simulink model "mrefrobotarm_modified_previous_y_previous_u_previous_ref"  (R2018b)
settings: Solver=FixedStepAuto  StartTime=0.0  StopTime=10  RelTol=1e-3  AbsTol=1e-6
undefined symbols (not defined in the file or in its folder): options, sfunxy2
libraries: neural x949, simulink x1
(part 12 of 31)

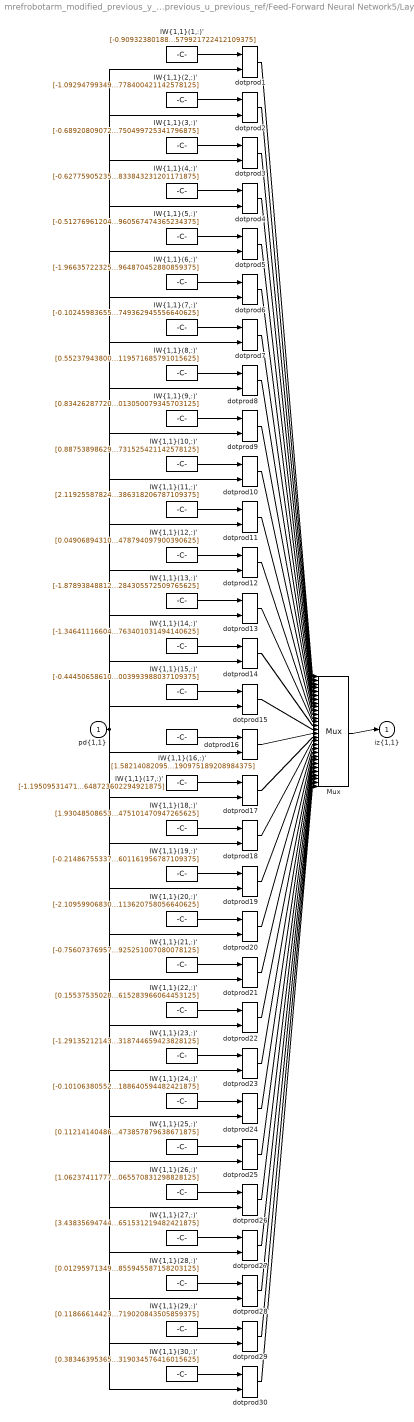
== system mrefrobotarm_modified_previous_y_previous_u_previous_ref/Feed-Forward Neural Network5/Layer 1/IW{1,1} ==
  "pd{1,1}" : Inport  PortDimensions=10
      mask Display: e = 0.06;c1 = [120 230 180]/255;c2 = ([120 230 180]+0)/(256+128);c3 = ([120 230 180]+128)/(256+128);patch([0 1 1 0],[0 0 1 1],c1);patch([0 1 1 1-e 1-e 0+e],[0 0 1 1-e 0+e 0+e],c2);patch([0 0 1 1-e 0+e 0+e],[0 1 1 1-e 1-e 0+e],c3);plot([0 1 1 0 0],[0 0 1 1 0]);
  "IW{1,1}(1,:)'" : Constant  Value=[-0.90932380188037520429844562386278994381427764892578125;0.76371033894988615831067590988823212683200836181640625;0.511083989829526519343971813214011490345001220703125;1.0944032703019865859772608018829487264156341552734375;0.0136695027619473281899065142397375893779098987579345703125;0.1974163924613260012730364678645855747163295745849609375;0.464743606324651781225298918798216618597507476806640625;-0.1561130566172034550564973187647410668432712554931640625;-0.5876780806125221356950305562349967658519744873046875;-0.323235939703412744616883855997002683579921722412109375]
      mask Display: e = 0.06;c1 = [120 150 230]/255;c2 = ([120 150 230]+0)/383;c3 = ([120 150 230]+128)/383;patch([0 1 1 0],[0 0 1 1],c1);patch([0 1 1 1-e 1-e 0+e],[0 0 1 1-e 0+e 0+e],c2);patch([0 0 1 1-e 0+e 0+e],[0 1 1 1-e 1-e 0+e],c3);plot([0 1 1 0 0],[0 0 1 1 0]);disp('Weights');
  "IW{1,1}(10,:)'" : Constant  Value=[0.887538986299241994260000865324400365352630615234375;-1.2998333260689995949377362194354645907878875732421875;0.6289189474694139025956474142731167376041412353515625;0.03883094077027136881152813430162495933473110198974609375;-0.63589794379239228394595784266130067408084869384765625;-0.146677513818444904547533269578707404434680938720703125;-0.313067428723999674478051247206167317926883697509765625;-0.0115715976737959906628372408476934651844203472137451171875;0.42402408377306699538422662953962571918964385986328125;0.1108860373607776228510601868038065731525421142578125]
      mask Display: e = 0.06;c1 = [120 150 230]/255;c2 = ([120 150 230]+0)/383;c3 = ([120 150 230]+128)/383;patch([0 1 1 0],[0 0 1 1],c1);patch([0 1 1 1-e 1-e 0+e],[0 0 1 1-e 0+e 0+e],c2);patch([0 0 1 1-e 0+e 0+e],[0 1 1 1-e 1-e 0+e],c3);plot([0 1 1 0 0],[0 0 1 1 0]);disp('Weights');
  "IW{1,1}(11,:)'" : Constant  Value=[2.119255878248722080314792037825100123882293701171875;-0.7549499748038221991208729377831332385540008544921875;-1.11661451283914647802930630859918892383575439453125;-0.398157577160634323920618271586135961115360260009765625;-1.13162667022485319279212490073405206203460693359375;0.80435012572452035950476556536159478127956390380859375;0.7029651111174974875694942966219969093799591064453125;-0.257844369723556621210036610136739909648895263671875;-0.1686892089893979040926552670498494990170001983642578125;-0.190349557734720453705534737309790216386318206787109375]
      mask Display: e = 0.06;c1 = [120 150 230]/255;c2 = ([120 150 230]+0)/383;c3 = ([120 150 230]+128)/383;patch([0 1 1 0],[0 0 1 1],c1);patch([0 1 1 1-e 1-e 0+e],[0 0 1 1-e 0+e 0+e],c2);patch([0 0 1 1-e 0+e 0+e],[0 1 1 1-e 1-e 0+e],c3);plot([0 1 1 0 0],[0 0 1 1 0]);disp('Weights');
  "IW{1,1}(12,:)'" : Constant  Value=[0.049068943101151452079733417122042737901210784912109375;-1.482782182940682869087822837173007428646087646484375;1.5668343168077765170664861216209828853607177734375;-0.318943372517797529841487857993342913687229156494140625;-0.545573934759136847105764900334179401397705078125;1.1430644568824648299454338484792970120906829833984375;-0.467368252058762478906572823689202778041362762451171875;-0.0230694534923694162531493390133618959225714206695556640625;0.07801593551157563755094059843031573109328746795654296875;0.0214066078871634514479982414059122675098478794097900390625]
      mask Display: e = 0.06;c1 = [120 150 230]/255;c2 = ([120 150 230]+0)/383;c3 = ([120 150 230]+128)/383;patch([0 1 1 0],[0 0 1 1],c1);patch([0 1 1 1-e 1-e 0+e],[0 0 1 1-e 0+e 0+e],c2);patch([0 0 1 1-e 0+e 0+e],[0 1 1 1-e 1-e 0+e],c3);plot([0 1 1 0 0],[0 0 1 1 0]);disp('Weights');
  "IW{1,1}(13,:)'" : Constant  Value=[-1.8789384881240140945379835102357901632785797119140625;3.441410048030609569735815966851077973842620849609375;-1.471086522236758842296922011882998049259185791015625;-0.14898768444497323404362987275817431509494781494140625;-0.399106474358735419105670416684006340801715850830078125;0.6532412791866761825332332591642625629901885986328125;-0.38852173803112322048036730848252773284912109375;0.0032598771438785306177321476894803709001280367374420166015625;-0.01042637952650987860636622173160503734834492206573486328125;0.101455793098639779348246747758821584284305572509765625]
      mask Display: e = 0.06;c1 = [120 150 230]/255;c2 = ([120 150 230]+0)/383;c3 = ([120 150 230]+128)/383;patch([0 1 1 0],[0 0 1 1],c1);patch([0 1 1 1-e 1-e 0+e],[0 0 1 1-e 0+e 0+e],c2);patch([0 0 1 1-e 0+e 0+e],[0 1 1 1-e 1-e 0+e],c3);plot([0 1 1 0 0],[0 0 1 1 0]);disp('Weights');
  "IW{1,1}(14,:)'" : Constant  Value=[-1.3464111660412154680699359232676215469837188720703125;-1.1074716408539320156023677554912865161895751953125;0.2010424729824872580596917259754263795912265777587890625;0.92341948049771682693886987181031145155429840087890625;1.246938309743069961399442036054097115993499755859375;0.01085945570533902553023164472278949688188731670379638671875;-0.81735505804402286411658451470430009067058563232421875;-0.1492403379165857801869066179278888739645481109619140625;-0.26249705798296785186352053642622195184230804443359375;-0.1124250257004068276334152187700965441763401031494140625]
      mask Display: e = 0.06;c1 = [120 150 230]/255;c2 = ([120 150 230]+0)/383;c3 = ([120 150 230]+128)/383;patch([0 1 1 0],[0 0 1 1],c1);patch([0 1 1 1-e 1-e 0+e],[0 0 1 1-e 0+e 0+e],c2);patch([0 0 1 1-e 0+e 0+e],[0 1 1 1-e 1-e 0+e],c3);plot([0 1 1 0 0],[0 0 1 1 0]);disp('Weights');
  "IW{1,1}(15,:)'" : Constant  Value=[-0.444506586108001811030732142171473242342472076416015625;-0.97492464854400318063909480770234949886798858642578125;-0.13235530416492380378912230298737995326519012451171875;0.041227831087679085719788218966641579754650592803955078125;0.302266181113509058153709929683827795088291168212890625;0.78147258701436339567436561992508359253406524658203125;-0.95056085210709528876549256892758421599864959716796875;-0.12105152846243098785361524960535462014377117156982421875;-0.25617381118761428648866740331868641078472137451171875;-0.1020694078831504147952813355004764162003993988037109375]
      mask Display: e = 0.06;c1 = [120 150 230]/255;c2 = ([120 150 230]+0)/383;c3 = ([120 150 230]+128)/383;patch([0 1 1 0],[0 0 1 1],c1);patch([0 1 1 1-e 1-e 0+e],[0 0 1 1-e 0+e 0+e],c2);patch([0 0 1 1-e 0+e 0+e],[0 1 1 1-e 1-e 0+e],c3);plot([0 1 1 0 0],[0 0 1 1 0]);disp('Weights');
  "IW{1,1}(16,:)'" : Constant  Value=[1.5821408209558025514951395962270908057689666748046875;-0.06572990373471408742656052481834194622933864593505859375;-0.315110468167437096642657934353337623178958892822265625;-0.546724857613621662011382795753888785839080810546875;0.6203138051412249165394996452960185706615447998046875;-0.313776979421296953187692224673810414969921112060546875;0.757180165723499332131041228421963751316070556640625;-0.54836876706250758939376055423053912818431854248046875;-0.701850548599278756256580891204066574573516845703125;-0.5565611120524296406841813222854398190975189208984375]
      mask Display: e = 0.06;c1 = [120 150 230]/255;c2 = ([120 150 230]+0)/383;c3 = ([120 150 230]+128)/383;patch([0 1 1 0],[0 0 1 1],c1);patch([0 1 1 1-e 1-e 0+e],[0 0 1 1-e 0+e 0+e],c2);patch([0 0 1 1-e 0+e 0+e],[0 1 1 1-e 1-e 0+e],c3);plot([0 1 1 0 0],[0 0 1 1 0]);disp('Weights');
  "IW{1,1}(17,:)'" : Constant  Value=[-1.1950953147174991908485708336229436099529266357421875;2.3757652564865896493984109838493168354034423828125;-0.38308523924205239996609861918841488659381866455078125;-0.96383528447031319164040041869156993925571441650390625;0.2203039003468626744197678135606111027300357818603515625;-0.497348839684495114266127302471431903541088104248046875;0.1697163099235504402084728781119338236749172210693359375;-0.04046984692262479976765376932235085405409336090087890625;0.2877799138689625113585179860820062458515167236328125;-0.232984678848339121781663152432884089648723602294921875]
      mask Display: e = 0.06;c1 = [120 150 230]/255;c2 = ([120 150 230]+0)/383;c3 = ([120 150 230]+128)/383;patch([0 1 1 0],[0 0 1 1],c1);patch([0 1 1 1-e 1-e 0+e],[0 0 1 1-e 0+e 0+e],c2);patch([0 0 1 1-e 0+e 0+e],[0 1 1 1-e 1-e 0+e],c3);plot([0 1 1 0 0],[0 0 1 1 0]);disp('Weights');
  "IW{1,1}(18,:)'" : Constant  Value=[1.930485086537676142626196451601572334766387939453125;-1.2072210605310542685941754825762473046779632568359375;-0.711007077704297163478486254462040960788726806640625;-0.2130863010885823694007257245175424031913280487060546875;-0.40379224197537089136034182956791482865810394287109375;1.7657478700875628430111419220338575541973114013671875;-1.5367708627335885385178926298976875841617584228515625;0.2230269588249802203971938752147252671420574188232421875;0.28436213533471310643818696917151100933551788330078125;0.565124166666441940520826392457820475101470947265625]
      mask Display: e = 0.06;c1 = [120 150 230]/255;c2 = ([120 150 230]+0)/383;c3 = ([120 150 230]+128)/383;patch([0 1 1 0],[0 0 1 1],c1);patch([0 1 1 1-e 1-e 0+e],[0 0 1 1-e 0+e 0+e],c2);patch([0 0 1 1-e 0+e 0+e],[0 1 1 1-e 1-e 0+e],c3);plot([0 1 1 0 0],[0 0 1 1 0]);disp('Weights');
  "IW{1,1}(19,:)'" : Constant  Value=[-0.21486755337977625490708533106953836977481842041015625;0.395584246940376804690941980879870243370532989501953125;-0.2253224646851052781482138698265771381556987762451171875;0.040212706119560938378132419757093884982168674468994140625;0.63784511537261978642021631458192132413387298583984375;1.05208490378944485854617596487514674663543701171875;-1.9098567669794672685412706414354033768177032470703125;-0.421676708484349571648408527835272252559661865234375;0.83670495443842762828268178054713644087314605712890625;0.371391406764616183178162600597715936601161956787109375]
      mask Display: e = 0.06;c1 = [120 150 230]/255;c2 = ([120 150 230]+0)/383;c3 = ([120 150 230]+128)/383;patch([0 1 1 0],[0 0 1 1],c1);patch([0 1 1 1-e 1-e 0+e],[0 0 1 1-e 0+e 0+e],c2);patch([0 0 1 1-e 0+e 0+e],[0 1 1 1-e 1-e 0+e],c3);plot([0 1 1 0 0],[0 0 1 1 0]);disp('Weights');
  "IW{1,1}(2,:)'" : Constant  Value=[-1.0929479934920554029531558626331388950347900390625;-0.9110333206059608723847986766486428678035736083984375;0.374121770485466853539691101104835979640483856201171875;-0.19106218415262887777572586855967529118061065673828125;-0.1366447102440979666226894551073201000690460205078125;0.5191466117199059482345546712167561054229736328125;0.006687993191504093548616083353408612310886383056640625;-0.86049560927963042455957065612892620265483856201171875;-0.997905267886916025332766366773284971714019775390625;-0.0924789369240235636926428242077236063778400421142578125]
      mask Display: e = 0.06;c1 = [120 150 230]/255;c2 = ([120 150 230]+0)/383;c3 = ([120 150 230]+128)/383;patch([0 1 1 0],[0 0 1 1],c1);patch([0 1 1 1-e 1-e 0+e],[0 0 1 1-e 0+e 0+e],c2);patch([0 0 1 1-e 0+e 0+e],[0 1 1 1-e 1-e 0+e],c3);plot([0 1 1 0 0],[0 0 1 1 0]);disp('Weights');
  "IW{1,1}(20,:)'" : Constant  Value=[-2.10959906830338272953895284445025026798248291015625;0.159367553973865760941208691292558796703815460205078125;1.8570827940161063196455870638601481914520263671875;-0.72380870444345346559344989145756699144840240478515625;-0.0092473189529538694919619246093134279362857341766357421875;0.283697195135588053904740490906988270580768585205078125;-0.5830490814708999547377743510878644883632659912109375;0.2075909773479038822330267066718079149723052978515625;-0.1952642709523432495988259915975504554808139801025390625;0.161618302484284159792338186889537610113620758056640625]
      mask Display: e = 0.06;c1 = [120 150 230]/255;c2 = ([120 150 230]+0)/383;c3 = ([120 150 230]+128)/383;patch([0 1 1 0],[0 0 1 1],c1);patch([0 1 1 1-e 1-e 0+e],[0 0 1 1-e 0+e 0+e],c2);patch([0 0 1 1-e 0+e 0+e],[0 1 1 1-e 1-e 0+e],c3);plot([0 1 1 0 0],[0 0 1 1 0]);disp('Weights');
  "IW{1,1}(21,:)'" : Constant  Value=[-0.75607376957241811954446575327892787754535675048828125;-0.485919162132690318767203052630065940320491790771484375;1.3296205299340291272613967521465383470058441162109375;-0.5149256369311785430653571893344633281230926513671875;-1.2990976297079879220319753585499711334705352783203125;0.21246699553293357798366969291237182915210723876953125;0.10428477162409578726798287107158103026449680328369140625;-0.344528308524458093398123992301407270133495330810546875;0.428403831244886845741604020076920278370380401611328125;0.038823305731819086894507364604578469879925251007080078125]
      mask Display: e = 0.06;c1 = [120 150 230]/255;c2 = ([120 150 230]+0)/383;c3 = ([120 150 230]+128)/383;patch([0 1 1 0],[0 0 1 1],c1);patch([0 1 1 1-e 1-e 0+e],[0 0 1 1-e 0+e 0+e],c2);patch([0 0 1 1-e 0+e 0+e],[0 1 1 1-e 1-e 0+e],c3);plot([0 1 1 0 0],[0 0 1 1 0]);disp('Weights');
  "IW{1,1}(22,:)'" : Constant  Value=[0.155375350285706204100932836809079162776470184326171875;-0.26459676100668938492077586488449014723300933837890625;-0.60328902141019480342976066822302527725696563720703125;0.70160472182963007359290941167273558676242828369140625;0.005274967361639301167974824835482650087215006351470947265625;-0.199857050065932018156900085159577429294586181640625;-0.88528258669875692365991426413529552519321441650390625;0.81731906964735456799786561532528139650821685791015625;1.0407361888036295027859523543156683444976806640625;0.451432794201563514224773143723723478615283966064453125]
      mask Display: e = 0.06;c1 = [120 150 230]/255;c2 = ([120 150 230]+0)/383;c3 = ([120 150 230]+128)/383;patch([0 1 1 0],[0 0 1 1],c1);patch([0 1 1 1-e 1-e 0+e],[0 0 1 1-e 0+e 0+e],c2);patch([0 0 1 1-e 0+e 0+e],[0 1 1 1-e 1-e 0+e],c3);plot([0 1 1 0 0],[0 0 1 1 0]);disp('Weights');
  "IW{1,1}(23,:)'" : Constant  Value=[-1.2913521214339349629796060980879701673984527587890625;0.050616472119993267952953175381480832584202289581298828125;-0.5153169585812984454520346844219602644443511962890625;0.6526118194760976987112144342972896993160247802734375;-0.1114752095402402887192039315777947194874286651611328125;-1.1256897347294037015075218732818029820919036865234375;0.76857380197294988821710148840793408453464508056640625;0.33086064957372041117622529782238416373729705810546875;-0.01304188699703218330683274217562939156778156757354736328125;0.043505160056315612948640847434944589622318744659423828125]
      mask Display: e = 0.06;c1 = [120 150 230]/255;c2 = ([120 150 230]+0)/383;c3 = ([120 150 230]+128)/383;patch([0 1 1 0],[0 0 1 1],c1);patch([0 1 1 1-e 1-e 0+e],[0 0 1 1-e 0+e 0+e],c2);patch([0 0 1 1-e 0+e 0+e],[0 1 1 1-e 1-e 0+e],c3);plot([0 1 1 0 0],[0 0 1 1 0]);disp('Weights');
  "IW{1,1}(24,:)'" : Constant  Value=[-0.10106380552618100809869616796277114190161228179931640625;-0.90711288404816226016436075951787643134593963623046875;-0.68833658988813295476205667000613175332546234130859375;0.1932642625719050155641554056273889727890491485595703125;0.9823876294081956839221447808085940778255462646484375;0.265523912386287086473402041519875638186931610107421875;-1.027465427708543099782900753780268132686614990234375;0.1170088921222139088929026229379815049469470977783203125;0.28734573897554460675252130386070348322391510009765625;0.43804995252470113609177815305883996188640594482421875]
      mask Display: e = 0.06;c1 = [120 150 230]/255;c2 = ([120 150 230]+0)/383;c3 = ([120 150 230]+128)/383;patch([0 1 1 0],[0 0 1 1],c1);patch([0 1 1 1-e 1-e 0+e],[0 0 1 1-e 0+e 0+e],c2);patch([0 0 1 1-e 0+e 0+e],[0 1 1 1-e 1-e 0+e],c3);plot([0 1 1 0 0],[0 0 1 1 0]);disp('Weights');
  "IW{1,1}(25,:)'" : Constant  Value=[0.11214140486703887134023460703247110359370708465576171875;-1.471506488355823538682898288243450224399566650390625;0.133531147598676735999134734811377711594104766845703125;1.122363315661508043064031880930997431278228759765625;1.28012792324946556021814103587530553340911865234375;-0.74237881431375274399186992013710550963878631591796875;0.66710183705330872161454180968576110899448394775390625;-0.70877060054504859021307083821739070117473602294921875;-0.485049297948819291281807863924768753349781036376953125;-0.1574484298191662912103083726833574473857879638671875]
      mask Display: e = 0.06;c1 = [120 150 230]/255;c2 = ([120 150 230]+0)/383;c3 = ([120 150 230]+128)/383;patch([0 1 1 0],[0 0 1 1],c1);patch([0 1 1 1-e 1-e 0+e],[0 0 1 1-e 0+e 0+e],c2);patch([0 0 1 1-e 0+e 0+e],[0 1 1 1-e 1-e 0+e],c3);plot([0 1 1 0 0],[0 0 1 1 0]);disp('Weights');
  "IW{1,1}(26,:)'" : Constant  Value=[1.0623741177703573956847549197846092283725738525390625;-0.6781159561656291412390373807284049689769744873046875;-0.443594968790031074501456487269024364650249481201171875;-0.43757504643029709878732091965503059327602386474609375;0.82842085740769821899931457664933986961841583251953125;-0.42101339044706731495892881866893731057643890380859375;-0.42136360919663740087770520403864793479442596435546875;-0.1496866336070057368345942450105212628841400146484375;-0.300316340034200990327661884293775074183940887451171875;-0.1785110450305303075868579298912663944065570831298828125]
      mask Display: e = 0.06;c1 = [120 150 230]/255;c2 = ([120 150 230]+0)/383;c3 = ([120 150 230]+128)/383;patch([0 1 1 0],[0 0 1 1],c1);patch([0 1 1 1-e 1-e 0+e],[0 0 1 1-e 0+e 0+e],c2);patch([0 0 1 1-e 0+e 0+e],[0 1 1 1-e 1-e 0+e],c3);plot([0 1 1 0 0],[0 0 1 1 0]);disp('Weights');
  "IW{1,1}(27,:)'" : Constant  Value=[3.438356947442843480899909991421736776828765869140625;-1.62061060946207202704272276605479419231414794921875;-1.2986020787082852567806412480422295629978179931640625;-0.53333605278638096525156697680358774960041046142578125;-0.00840598569886454038968537361142807640135288238525390625;-1.4060867563995473883409204063354991376399993896484375;0.5859728532113035459616412481409497559070587158203125;0.275323908043609899554127196097397245466709136962890625;0.0182615390406305200254877263432717882096767425537109375;-0.14015911457563212660915041851694695651531219482421875]
      mask Display: e = 0.06;c1 = [120 150 230]/255;c2 = ([120 150 230]+0)/383;c3 = ([120 150 230]+128)/383;patch([0 1 1 0],[0 0 1 1],c1);patch([0 1 1 1-e 1-e 0+e],[0 0 1 1-e 0+e 0+e],c2);patch([0 0 1 1-e 0+e 0+e],[0 1 1 1-e 1-e 0+e],c3);plot([0 1 1 0 0],[0 0 1 1 0]);disp('Weights');
  "IW{1,1}(28,:)'" : Constant  Value=[0.01295971349550303040876197968600536114536225795745849609375;0.56009597191418070138979601324535906314849853515625;0.69838391643163266753191464886185713112354278564453125;0.1536338633683131948970412850030697882175445556640625;-1.48212155227424613457287705386988818645477294921875;0.1500202134438412826522579734955797903239727020263671875;0.89614815972182093606335229196702130138874053955078125;-0.153300578840785239886912449946976266801357269287109375;-0.86809858066474243631915896912687458097934722900390625;-0.66052662099663461692244936784845776855945587158203125]
      mask Display: e = 0.06;c1 = [120 150 230]/255;c2 = ([120 150 230]+0)/383;c3 = ([120 150 230]+128)/383;patch([0 1 1 0],[0 0 1 1],c1);patch([0 1 1 1-e 1-e 0+e],[0 0 1 1-e 0+e 0+e],c2);patch([0 0 1 1-e 0+e 0+e],[0 1 1 1-e 1-e 0+e],c3);plot([0 1 1 0 0],[0 0 1 1 0]);disp('Weights');
  "IW{1,1}(29,:)'" : Constant  Value=[0.11866614423466127770101508076550089754164218902587890625;-0.440042241888271179472980065838783048093318939208984375;0.267582889104284460390914546223939396440982818603515625;0.804731306823940339967293766676448285579681396484375;0.69374030400950648100888429326005280017852783203125;-0.752193514755144843064726956072263419628143310546875;-0.47951825292688521340522811442497186362743377685546875;0.19184747725769124571115753496997058391571044921875;-1.0662089218825894221254202420823276042938232421875;-0.33084984051937949001143124405643902719020843505859375]
      mask Display: e = 0.06;c1 = [120 150 230]/255;c2 = ([120 150 230]+0)/383;c3 = ([120 150 230]+128)/383;patch([0 1 1 0],[0 0 1 1],c1);patch([0 1 1 1-e 1-e 0+e],[0 0 1 1-e 0+e 0+e],c2);patch([0 0 1 1-e 0+e 0+e],[0 1 1 1-e 1-e 0+e],c3);plot([0 1 1 0 0],[0 0 1 1 0]);disp('Weights');
  "IW{1,1}(3,:)'" : Constant  Value=[-0.6892080907265862865784811219782568514347076416015625;-0.295383977713851997304317364978487603366374969482421875;0.25580863769639450300275029803742654621601104736328125;0.75887860793579153817489668654161505401134490966796875;0.340850039499524359865034739414113573729991912841796875;0.97377565386021724957998912941548041999340057373046875;-0.007272230474530954648371139370510718435980379581451416015625;-0.88085798295643835675861055278801359236240386962890625;0.2720192458025765258611272656708024442195892333984375;0.0022109667407200074389084232251434514182619750499725341796875]
      mask Display: e = 0.06;c1 = [120 150 230]/255;c2 = ([120 150 230]+0)/383;c3 = ([120 150 230]+128)/383;patch([0 1 1 0],[0 0 1 1],c1);patch([0 1 1 1-e 1-e 0+e],[0 0 1 1-e 0+e 0+e],c2);patch([0 0 1 1-e 0+e 0+e],[0 1 1 1-e 1-e 0+e],c3);plot([0 1 1 0 0],[0 0 1 1 0]);disp('Weights');
  "IW{1,1}(30,:)'" : Constant  Value=[0.383463953650225841673915283536189235746860504150390625;-0.520489063876894864080213665147311985492706298828125;-0.20966583834922192242089522551395930349826812744140625;0.2312684491234270611759171742960461415350437164306640625;0.0631731969837025231218063936466933228075504302978515625;-1.247839828748543045122687544790096580982208251953125;-0.6484077584290768303532104255282320082187652587890625;0.701602364259750199693144168122671544551849365234375;0.040912301585527728609026354433808592148125171661376953125;-0.183953638197987656699439185103983618319034576416015625]
      mask Display: e = 0.06;c1 = [120 150 230]/255;c2 = ([120 150 230]+0)/383;c3 = ([120 150 230]+128)/383;patch([0 1 1 0],[0 0 1 1],c1);patch([0 1 1 1-e 1-e 0+e],[0 0 1 1-e 0+e 0+e],c2);patch([0 0 1 1-e 0+e 0+e],[0 1 1 1-e 1-e 0+e],c3);plot([0 1 1 0 0],[0 0 1 1 0]);disp('Weights');
  "IW{1,1}(4,:)'" : Constant  Value=[-0.6277590523507503572631094357348047196865081787109375;-0.52277551306430958266702191394870169460773468017578125;0.87244686961718687090439061648794449865818023681640625;0.38191906652647633624297895948984660208225250244140625;0.329967024944724018897801443017669953405857086181640625;-1.1831597365391364196085532967117615044116973876953125;0.6718701186851647744191495803534053266048431396484375;-0.09039670806665102420485169432140537537634372711181640625;0.51395514831622179929837557210703380405902862548828125;-0.3885004765678317095733973474125377833843231201171875]
      mask Display: e = 0.06;c1 = [120 150 230]/255;c2 = ([120 150 230]+0)/383;c3 = ([120 150 230]+128)/383;patch([0 1 1 0],[0 0 1 1],c1);patch([0 1 1 1-e 1-e 0+e],[0 0 1 1-e 0+e 0+e],c2);patch([0 0 1 1-e 0+e 0+e],[0 1 1 1-e 1-e 0+e],c3);plot([0 1 1 0 0],[0 0 1 1 0]);disp('Weights');
  "IW{1,1}(5,:)'" : Constant  Value=[-0.51276961204605708832815480491262860596179962158203125;-0.61638799657158427347525275763473473489284515380859375;-0.43041893732653824233835848644957877695560455322265625;-0.5678563219639183312636987466248683631420135498046875;0.71295871833810464668346185135305859148502349853515625;0.5069882237113041423270942686940543353557586669921875;-0.771365526256594602472205224330537021160125732421875;-0.647214466957101830502097072894684970378875732421875;-0.39165850392566292637042124624713324010372161865234375;0.36692561849499705228794255162938497960567474365234375]
      mask Display: e = 0.06;c1 = [120 150 230]/255;c2 = ([120 150 230]+0)/383;c3 = ([120 150 230]+128)/383;patch([0 1 1 0],[0 0 1 1],c1);patch([0 1 1 1-e 1-e 0+e],[0 0 1 1-e 0+e 0+e],c2);patch([0 0 1 1-e 0+e 0+e],[0 1 1 1-e 1-e 0+e],c3);plot([0 1 1 0 0],[0 0 1 1 0]);disp('Weights');
  "IW{1,1}(6,:)'" : Constant  Value=[-1.9663572232534107797619071789085865020751953125;-0.11268110413806649294787831649955478496849536895751953125;1.109073141398012385394622469902969896793365478515625;1.010454381619202646191979511058889329433441162109375;1.2454755259900494035463225372950546443462371826171875;-1.2244803494318470260537878857576288282871246337890625;0.47575372335666354928207510965876281261444091796875;-0.032169783249202645036834979919149191118776798248291015625;-0.11798391234503312341441727539859130047261714935302734375;-0.0990151297793054607776497277882299385964870452880859375]
      mask Display: e = 0.06;c1 = [120 150 230]/255;c2 = ([120 150 230]+0)/383;c3 = ([120 150 230]+128)/383;patch([0 1 1 0],[0 0 1 1],c1);patch([0 1 1 1-e 1-e 0+e],[0 0 1 1-e 0+e 0+e],c2);patch([0 0 1 1-e 0+e 0+e],[0 1 1 1-e 1-e 0+e],c3);plot([0 1 1 0 0],[0 0 1 1 0]);disp('Weights');
  "IW{1,1}(7,:)'" : Constant  Value=[-0.10245983655072689322285128810108290053904056549072265625;0.25978944641103607349208459709188900887966156005859375;1.112199661826462016023242540541104972362518310546875;0.04289802162162702214853737814337364397943019866943359375;-0.06838647702837967468081359356801840476691722869873046875;-0.2089553652550784068608891175244934856891632080078125;1.0901624896618182791740991888218559324741363525390625;-0.497477970022246418491107533554895780980587005615234375;-0.13781908983157042936085190376616083085536956787109375;-0.3812135547315025352332895636209286749362945556640625]
      mask Display: e = 0.06;c1 = [120 150 230]/255;c2 = ([120 150 230]+0)/383;c3 = ([120 150 230]+128)/383;patch([0 1 1 0],[0 0 1 1],c1);patch([0 1 1 1-e 1-e 0+e],[0 0 1 1-e 0+e 0+e],c2);patch([0 0 1 1-e 0+e 0+e],[0 1 1 1-e 1-e 0+e],c3);plot([0 1 1 0 0],[0 0 1 1 0]);disp('Weights');
  "IW{1,1}(8,:)'" : Constant  Value=[0.5523794380031354922522268680040724575519561767578125;-0.1643062236496783956596345888101495802402496337890625;-0.63177104006039552785978230531327426433563232421875;-0.73591572388689396877481385672581382095813751220703125;-0.206427314148784180058981974070775322616100311279296875;-0.01378706403715858862246701477261012769304215908050537109375;0.1393973915830730714304763750988058745861053466796875;-0.65212806505696629955082244123332202434539794921875;0.64843378131981210810153015700052492320537567138671875;-0.08479896804780885644081678265138179995119571685791015625]
      mask Display: e = 0.06;c1 = [120 150 230]/255;c2 = ([120 150 230]+0)/383;c3 = ([120 150 230]+128)/383;patch([0 1 1 0],[0 0 1 1],c1);patch([0 1 1 1-e 1-e 0+e],[0 0 1 1-e 0+e 0+e],c2);patch([0 0 1 1-e 0+e 0+e],[0 1 1 1-e 1-e 0+e],c3);plot([0 1 1 0 0],[0 0 1 1 0]);disp('Weights');
  "IW{1,1}(9,:)'" : Constant  Value=[0.83426287720403358161291862415964715182781219482421875;-0.92694728314541008362681395738036371767520904541015625;1.0158274178284296684893206474953331053256988525390625;-0.7719317073072053947413451169268228113651275634765625;0.041236082570084979515012690853836829774081707000732421875;0.10884898696354437797051417646798654459416866302490234375;-0.318593310561415210546698517646291293203830718994140625;0.0356863837331576616573869387138984166085720062255859375;0.65333173369441244204836038989014923572540283203125;-0.0945891743479452540288576756211114116013050079345703125]
      mask Display: e = 0.06;c1 = [120 150 230]/255;c2 = ([120 150 230]+0)/383;c3 = ([120 150 230]+128)/383;patch([0 1 1 0],[0 0 1 1],c1);patch([0 1 1 1-e 1-e 0+e],[0 0 1 1-e 0+e 0+e],c2);patch([0 0 1 1-e 0+e 0+e],[0 1 1 1-e 1-e 0+e],c3);plot([0 1 1 0 0],[0 0 1 1 0]);disp('Weights');
  Mux : Mux  Inputs=30
      mask Display: e = 0.06;c1 = [120 150 230]/255;c2 = ([120 150 230]+0)/383;c3 = ([120 150 230]+128)/383;patch([0 1 1 0],[0 0 1 1],c1);patch([0 1 1 1-e 1-e 0+e],[0 0 1 1-e 0+e 0+e],c2);patch([0 0 1 1-e 0+e 0+e],[0 1 1 1-e 1-e 0+e],c3);plot([0 1 1 0 0],[0 0 1 1 0]);disp('Mux');
  dotprod{1..30} (30 alike) : neural/Weight Functions/dotprod
  "iz{1,1}" : Outport
      mask Display: e = 0.06;c1 = [120 230 180]/255;c2 = ([120 230 180]+0)/(256+128);c3 = ([120 230 180]+128)/(256+128);patch([0 1 1 0],[0 0 1 1],c1);patch([0 1 1 1-e 1-e 0+e],[0 0 1 1-e 0+e 0+e],c2);patch([0 0 1 1-e 0+e 0+e],[0 1 1 1-e 1-e 0+e],c3);plot([0 1 1 0 0],[0 0 1 1 0]);
  wires:
  "IW{1,1}(1,:)'"/1 -> dotprod1/1
  "pd{1,1}"/1 -> dotprod1/2, dotprod2/2, dotprod3/2, dotprod4/2, dotprod5/2, dotprod6/2, dotprod7/2, dotprod8/2, dotprod9/2, dotprod10/2, dotprod11/2, dotprod12/2, dotprod13/2, dotprod14/2, dotprod15/2, dotprod16/2, dotprod17/2, dotprod18/2, dotprod19/2, dotprod20/2, dotprod21/2, dotprod22/2, dotprod23/2, dotprod24/2, dotprod25/2, dotprod26/2, dotprod27/2, dotprod28/2, dotprod29/2, dotprod30/2
  dotprod1/1 -> Mux/1
  "IW{1,1}(2,:)'"/1 -> dotprod2/1
  dotprod2/1 -> Mux/2
  "IW{1,1}(3,:)'"/1 -> dotprod3/1
  dotprod3/1 -> Mux/3
  "IW{1,1}(4,:)'"/1 -> dotprod4/1
  dotprod4/1 -> Mux/4
  "IW{1,1}(5,:)'"/1 -> dotprod5/1
  dotprod5/1 -> Mux/5
  "IW{1,1}(6,:)'"/1 -> dotprod6/1
  dotprod6/1 -> Mux/6
  "IW{1,1}(7,:)'"/1 -> dotprod7/1
  dotprod7/1 -> Mux/7
  "IW{1,1}(8,:)'"/1 -> dotprod8/1
  dotprod8/1 -> Mux/8
  "IW{1,1}(9,:)'"/1 -> dotprod9/1
  dotprod9/1 -> Mux/9
  "IW{1,1}(10,:)'"/1 -> dotprod10/1
  dotprod10/1 -> Mux/10
  "IW{1,1}(11,:)'"/1 -> dotprod11/1
  dotprod11/1 -> Mux/11
  "IW{1,1}(12,:)'"/1 -> dotprod12/1
  dotprod12/1 -> Mux/12
  "IW{1,1}(13,:)'"/1 -> dotprod13/1
  dotprod13/1 -> Mux/13
  "IW{1,1}(14,:)'"/1 -> dotprod14/1
  dotprod14/1 -> Mux/14
  "IW{1,1}(15,:)'"/1 -> dotprod15/1
  dotprod15/1 -> Mux/15
  "IW{1,1}(16,:)'"/1 -> dotprod16/1
  dotprod16/1 -> Mux/16
  "IW{1,1}(17,:)'"/1 -> dotprod17/1
  dotprod17/1 -> Mux/17
  "IW{1,1}(18,:)'"/1 -> dotprod18/1
  dotprod18/1 -> Mux/18
  "IW{1,1}(19,:)'"/1 -> dotprod19/1
  dotprod19/1 -> Mux/19
  "IW{1,1}(20,:)'"/1 -> dotprod20/1
  dotprod20/1 -> Mux/20
  "IW{1,1}(21,:)'"/1 -> dotprod21/1
  dotprod21/1 -> Mux/21
  "IW{1,1}(22,:)'"/1 -> dotprod22/1
  dotprod22/1 -> Mux/22
  "IW{1,1}(23,:)'"/1 -> dotprod23/1
  dotprod23/1 -> Mux/23
  "IW{1,1}(24,:)'"/1 -> dotprod24/1
  dotprod24/1 -> Mux/24
  "IW{1,1}(25,:)'"/1 -> dotprod25/1
  dotprod25/1 -> Mux/25
  "IW{1,1}(26,:)'"/1 -> dotprod26/1
  dotprod26/1 -> Mux/26
  "IW{1,1}(27,:)'"/1 -> dotprod27/1
  dotprod27/1 -> Mux/27
  "IW{1,1}(28,:)'"/1 -> dotprod28/1
  dotprod28/1 -> Mux/28
  "IW{1,1}(29,:)'"/1 -> dotprod29/1
  dotprod29/1 -> Mux/29
  "IW{1,1}(30,:)'"/1 -> dotprod30/1
  dotprod30/1 -> Mux/30
  Mux/1 -> "iz{1,1}"/1

== system mrefrobotarm_modified_previous_y_previous_u_previous_ref/Feed-Forward Neural Network5/Layer 2/Delays 1 ==
  "p{2}" : Inport  PortDimensions=30
      mask Display: e = 0.06;c1 = [120 230 180]/255;c2 = ([120 230 180]+0)/(256+128);c3 = ([120 230 180]+128)/(256+128);patch([0 1 1 0],[0 0 1 1],c1);patch([0 1 1 1-e 1-e 0+e],[0 0 1 1-e 0+e 0+e],c2);patch([0 0 1 1-e 0+e 0+e],[0 1 1 1-e 1-e 0+e],c3);plot([0 1 1 0 0],[0 0 1 1 0]);
  mux : Mux  Inputs=1
      mask Display: e = 0.06;c1 = [120 150 230]/255;c2 = ([120 150 230]+0)/383;c3 = ([120 150 230]+128)/383;patch([0 1 1 0],[0 0 1 1],c1);patch([0 1 1 1-e 1-e 0+e],[0 0 1 1-e 0+e 0+e],c2);patch([0 0 1 1-e 0+e 0+e],[0 1 1 1-e 1-e 0+e],c3);plot([0 1 1 0 0],[0 0 1 1 0]);disp('Mux')
  "pd{2,1}" : Outport
      mask Display: e = 0.06;c1 = [120 230 180]/255;c2 = ([120 230 180]+0)/(256+128);c3 = ([120 230 180]+128)/(256+128);patch([0 1 1 0],[0 0 1 1],c1);patch([0 1 1 1-e 1-e 0+e],[0 0 1 1-e 0+e 0+e],c2);patch([0 0 1 1-e 0+e 0+e],[0 1 1 1-e 1-e 0+e],c3);plot([0 1 1 0 0],[0 0 1 1 0]);
  wires:
  "p{2}"/1 -> mux/1
  mux/1 -> "pd{2,1}"/1
